simulink model "hw5q2"  (R2023b)
settings: Solver=VariableStepAuto  StartTime=0.0  StopTime=50  RelTol=1e-3
settings Model: Creator=vivek  LastModifiedBy=vivek

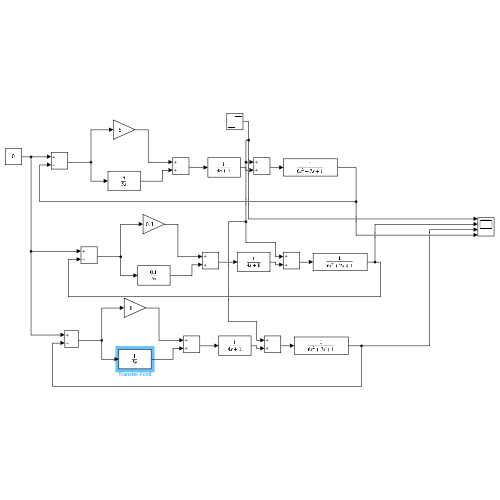
[thumbnail: Simulink's stored preview of the top-level diagram]
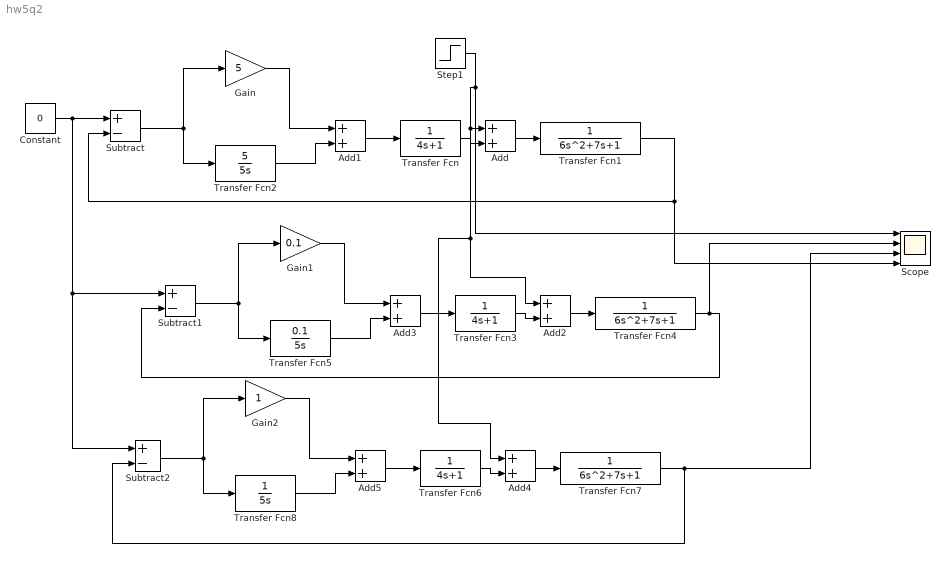
== system hw5q2 ==
  Add{,1..5} (6 alike) : Sum
  Constant : Constant  Value=0
  Gain : Gain  Gain=5
  Gain1 : Gain  Gain=0.1
  Gain2 : Gain
  Scope : Scope  NumInputPorts=4
  Step1 : Step  SampleTime=0
  Subtract : Sum  Inputs=+-
  Subtract1 : Sum  Inputs=+-
  Subtract2 : Sum  Inputs=+-
  Transfer Fcn : TransferFcn  Denominator=[4 1]
  Transfer Fcn1 : TransferFcn  Denominator=[6 7 1]
  Transfer Fcn2 : TransferFcn  Numerator=[5]  Denominator=[5 0]
  Transfer Fcn3 : TransferFcn  Denominator=[4 1]
  Transfer Fcn4 : TransferFcn  Denominator=[6 7 1]
  Transfer Fcn5 : TransferFcn  Numerator=[0.1]  Denominator=[5 0]
  Transfer Fcn6 : TransferFcn  Denominator=[4 1]
  Transfer Fcn7 : TransferFcn  Denominator=[6 7 1]
  Transfer Fcn8 : TransferFcn  Denominator=[5 0]
  wires:
  Gain/1 -> Add1/1
  Transfer Fcn1/1 -> Scope/4, Subtract/2
  Subtract/1 -> Transfer Fcn2/1, Gain/1
  Constant/1 -> Subtract2/1, Subtract1/1, Subtract/1
  Add/1 -> Transfer Fcn1/1
  Transfer Fcn/1 -> Add/2
  Transfer Fcn2/1 -> Add1/2
  Add1/1 -> Transfer Fcn/1
  Add3/1 -> Transfer Fcn3/1
  Transfer Fcn3/1 -> Add2/2
  Transfer Fcn5/1 -> Add3/2
  Subtract1/1 -> Gain1/1, Transfer Fcn5/1
  Gain1/1 -> Add3/1
  Add2/1 -> Transfer Fcn4/1
  Transfer Fcn4/1 -> Scope/2, Subtract1/2
  Subtract2/1 -> Gain2/1, Transfer Fcn8/1
  Gain2/1 -> Add5/1
  Add4/1 -> Transfer Fcn7/1
  Add5/1 -> Transfer Fcn6/1
  Transfer Fcn8/1 -> Add5/2
  Step1/1 -> Scope/1, Add4/1, Add2/1, Add/1
  Transfer Fcn6/1 -> Add4/2
  Transfer Fcn7/1 -> Subtract2/2, Scope/3
